simulink model "SIMULACION_FALANGE_PROXIMAL"  (Simulink 7.7)
settings: Solver=ode45  StartTime=0.0  StopTime=inf  RelTol=1e-3
libraries: simulink x2
settings Model: Creator=JohnConstantine  LastModifiedBy=JohnConstantine

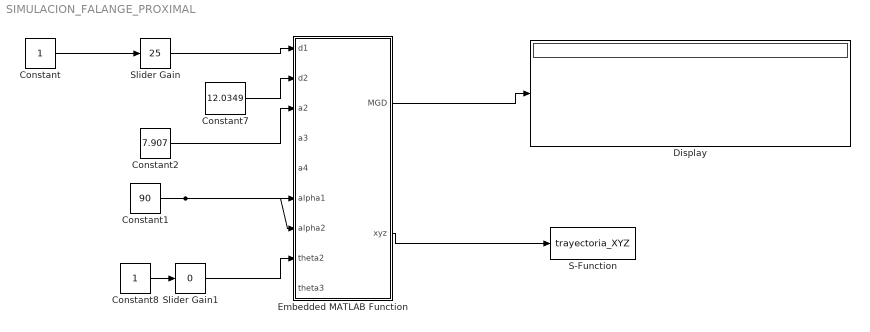
== system SIMULACION_FALANGE_PROXIMAL ==
  Constant : Constant
  Constant1 : Constant  Value=90
  Constant2 : Constant  Value=7.907
  Constant7 : Constant  Value=12.0349
  Constant8 : Constant
  Display : Display
  Embedded MATLAB Function : Stateflow chart  TreatAsAtomicUnit=on
  S-Function : S-Function  FunctionName=trayectoria_XYZ  Parameters=[-100 100 -100 100 -100 100]  EnableBusSupport=off
  Slider Gain : simulink/Math Operations/Slider Gain  SystemSampleTime=-1  low=0  gain=25  high=25
  Slider Gain1 : simulink/Math Operations/Slider Gain  SystemSampleTime=-1  low=0  gain=0  high=15
  wires:
  Constant/1 -> Slider Gain/1
  Constant1/1 -> Embedded MATLAB Function/6(alpha1), Embedded MATLAB Function/7(alpha2)
  Constant2/1 -> Embedded MATLAB Function/3(a2)
  Slider Gain/1 -> Embedded MATLAB Function/1(d1)
  Constant8/1 -> Slider Gain1/1
  Slider Gain1/1 -> Embedded MATLAB Function/8(theta2)
  Embedded MATLAB Function/1(MGD) -> Display/1
  Embedded MATLAB Function/2(xyz) -> S-Function/1
  Constant7/1 -> Embedded MATLAB Function/2(d2)

== matlab function Embedded MATLAB Function ==
  data: d1 input double; MGD output double; d2 input double; a2 input double; a3 input double; a4 input double; alpha1 input double; alpha2 input double; theta2 input double; xyz output double; theta3 input double
function [MGD,xyz] =mgdFalange(d1,d2,a2,a3,a4,alpha1,alpha2,theta2,theta3)
                                                                
                                                             
MGD=[                                              cosd(theta2)*cosd(theta3) - cosd(alpha2)*sind(theta2)*sind(theta3),                                                     - cosd(theta2)*sind(theta3) - cosd(alpha2)*cosd(theta3)*sind(theta2),                                         sind(alpha2)*sind(theta2),                                                                                       cosd(theta2)*(a2 + d1) + cosd(theta2)*cosd(theta3)*(a3 + a4) - cosd(alpha2)*sind(theta2)*sind(theta3)*(a3 + a4);...
 cosd(alpha1)*cosd(theta3)*sind(theta2) - sind(theta3)*(sind(alpha1)*sind(alpha2) - cosd(alpha1)*cosd(alpha2)*cosd(theta2)), - cosd(theta3)*(sind(alpha1)*sind(alpha2) - cosd(alpha1)*cosd(alpha2)*cosd(theta2)) - cosd(alpha1)*sind(theta2)*sind(theta3), - cosd(alpha2)*sind(alpha1) - cosd(alpha1)*sind(alpha2)*cosd(theta2),      cosd(alpha1)*sind(theta2)*(a2 + d1) - d2*sind(alpha1) - sind(theta3)*(a3 + a4)*(sind(alpha1)*sind(alpha2) - cosd(alpha1)*cosd(alpha2)*cosd(theta2)) + cosd(alpha1)*cosd(theta3)*sind(theta2)*(a3 + a4);...
 sind(theta3)*(cosd(alpha1)*sind(alpha2) + cosd(alpha2)*sind(alpha1)*cosd(theta2)) + sind(alpha1)*cosd(theta3)*sind(theta2),   cosd(theta3)*(cosd(alpha1)*sind(alpha2) + cosd(alpha2)*sind(alpha1)*cosd(theta2)) - sind(alpha1)*sind(theta2)*sind(theta3),   cosd(alpha1)*cosd(alpha2) - sind(alpha1)*sind(alpha2)*cosd(theta2), d1 + d2*cosd(alpha1) + sind(alpha1)*sind(theta2)*(a2 + d1) + sind(theta3)*(a3 + a4)*(cosd(alpha1)*sind(alpha2) + cosd(alpha2)*sind(alpha1)*cosd(theta2)) + sind(alpha1)*cosd(theta3)*sind(theta2)*(a3 + a4);...
                                                                                                                 0,                                                                                                                   0,                                                               0,                                                                                                                                                                                               1]

xyz=[MGD(1,4) MGD(2,4) MGD(3,4)];
